simulink library "Flex_Cantilever_Lib"  (R2019b)
settings: Solver=ode45  StartTime=0.0  StopTime=10.0  RelTol=1e-3
undefined symbols (not defined in the file): cantilever_aluminum, fBeamElement, gcbh, mech_rtmsupport, mech_support
libraries: mblibv1 x11, Flex_Cantilever_Element_Lib x9, cstblocks x1, $bdroot x1, SingleDofForceElement x1
Description:
  | Copyright 2009-2017 The MathWorks, Inc. MathWorks, Inc.
settings Model: Creator=smiller  LastModifiedBy=bhisma
settings DataIOCC: LimitDataPoints=on  SaveFormat=Array  SignalLoggingSaveFormat=ModelDataLogs  ReturnWorkspaceOutputs=off
settings OptimizationCC: BlockReduction=off  BooleanDataType=off  ExpressionDepthLimit=2147483647  LifeSpan=inf
settings DebuggingCC: SaveWithParameterizedLinksMsg=none  UnderspecifiedInitializationDetection=Classic  MergeDetectMultiDrivingBlocksExec=none  SignalResolutionControl=TryResolveAllWithWarning  FcnCallInpInsideContextMsg=warning  AllowSymbolicDim=off  StateNameClashWarn=warning  SFUnexpectedBacktrackingDiag=warning  SFNoUnconditionalDefaultTransitionDiag=warning  SFExecutionAtInitializationDiag=none  ArithmeticOperatorsInVariantConditions=warning
settings HardwareCC: ProdBitPerPointer=32  ProdBitPerSizeT=32  ProdBitPerPtrDiffT=32  ProdLargestAtomicFloat=None  ProdIntDivRoundTo=Undefined  ProdEndianess=Unspecified  ProdWordSize=32  ProdHWDeviceType=32-bit Generic  TargetUnknown=on
settings ModelReferenceCC: PropagateSignalLabelsOutOfModel=off
settings SFSimCC: SimUseLocalCustomCode=off  CustomCodeUndefinedFunction=UseInterfaceOnly
settings RTWCC: RTWUseLocalCustomCode=off
settings CodeAppCC: StateflowObjectComments=on
settings GRTTargetCC: TargetLangStandard=C89/C90 (ANSI)  GeneratePreprocessorConditionals=Disable all  CombineOutputUpdateFcns=off  GRTInterface=on
settings ConfigComp: CovMetricSettings=dw  CovHtmlReporting=on  CovSaveCumulativeToWorkspaceVar=on  CovSaveSingleToWorkspaceVar=on  CovExternalEMLEnable=off  CovSFcnEnable=off

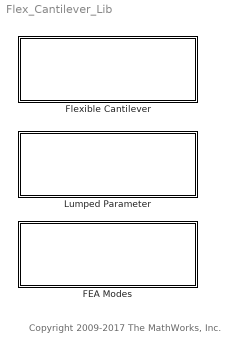
== system Flex_Cantilever_Lib ==
  note: Copyright 2009-2017 The MathWorks, Inc.
  FEA Modes : Subsystem  mask(Cantilever){cantileverData=cantilever_aluminum}
      mask prompts: cantileverData "Cantilever specification"
      mask help:
      | Models a rectangular cross-section cantilever.
      |
      | Specify the name of a cantilever data structure that has the following fields:
      | 	length
      | 	height
      | 	width
      | 	material.density
      | 	material.youngsModulus
      mask init:
      | derivedData = ...
      |     derive_cantilever_properties( cantileverData );
      | L        = derivedData.L;
      | a        = derivedData.a;
      | b        = derivedData.b;
      | volume   = derivedData.volume;
      | mass     = derivedData.mass;
      | inertia  = derivedData.inertia;
      mask Display: image(imread('Flexible_Cantilever_FEA_Beam_IMAGE.jpg'));
  Flexible Cantilever : Subsystem  BlockChoice=FEA Modes
      settings: TemplateBlock=self  MemberBlocks=FEA Modes,Lumped Parameter
  Lumped Parameter : Subsystem
      mask Display: image(imread('Flexible_Cantilever_Lumped_Parameter_IMAGE.jpg'));

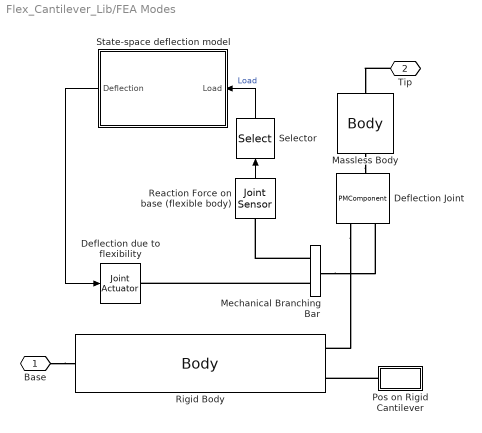
== system Flex_Cantilever_Lib/FEA Modes ==
  Deflection Joint : PMComponent  DialogController=MECH.DynMechDlgSource  LoadFcn=mech_rtmsupport('LoadFcn',gcbh);mech_support('LoadFcn',gcbh);  InitFcn=mech_support('InitFcn');  StartFcn=mech_support('StartFcn',gcbh);  StopFcn=mech_support('StopFcn',gcbh);  PhysicalDomain=mechanical  SubClassName=Unknown  LConnTagsString=__newl0|SA1  RConnTagsString=__newr0  mask(Prismatic){PMImportedID=, NumSAPorts=1, CutJoint=off, MarkAsCut=off, Primitives=prismatic, PrimitiveProps=P1$Base$[0 1 0]$prismatic, ClassName=Joint, DialogClass=JointBlock, P1Axis=[0 1 0]}
      mask prompts: PMImportedID "PMIMPORTED_ID"
      mask help: Represents one translational degree of freedom. The follower (F) body translates relative to the base (B) Body along single translational axis connecting Body coordinate origins. Sensor and actuator ports can be added. Base-follower sequence and axis direction determine sign of forward motion.
      mask init:
      | mech_preinitmask ();
      settings: CopyFcn=mech_rtmsupport('CopyFcn',gcbh);mech_support('CopyFcn',gcbh);  DeleteFcn=mech_rtmsupport('DeleteFcn',gcbh);mech_support('DeleteFcn',gcbh);  UndoDeleteFcn=mech_support('UndoDeleteFcn',gcbh);  ModelCloseFcn=mech_support('ModelCloseFcn',gcbh);  PreSaveFcn=mech_rtmsupport('PreSaveFcn',gcbh);mech_support('PreSaveFcn');  PostSaveFcn=mech_rtmsupport('PostSaveFcn',gcbh);mech_support('PostSaveFcn');  NameChangeFcn=mech_support('NameChangeFcn',gcbh);  PreCopyFcn=mech_rtmsupport('PreCopyFcn',gcbh);  CloseFcn=mech_support('CloseFcn',gcbh);  PreDeleteFcn=mech_rtmsupport('PreDeleteFcn',gcbh);
      mask Help: web(mech_help('prismatic'))
      mask Display: image(mech_getIcon('prismatic.bmp', 'Mechanical'),'center');color('red');text(mech_cutAffordance('offset', gcbh) - 2, 0, mech_cutAffordance('text', gcbh),'HorizontalAlignment', 'right','VerticalAlignment', 'bottom');color('magenta');port_label('LConn', 1, 'B');port_label('RConn', 1, 'F');
  Deflection due to flexibility : mblibv1/Sensors &  Actuators/Joint Actuator  UpdateFromCAD=off  PhysicalDomain=Mechanical  PortType=blob  ActuationStyle=Motion  AngleUnits=deg  ArcVelocityUnits=deg/s  ArcAccelerationUnits=deg/s^2  CoordPositionUnits=m  VelocityUnits=m/s  AccelerationUnits=m/s^2  ForceUnits=N  TorqueUnits=N*m  ActiveIO=off  Width=1  DialogClass=MechanicalActuatorBlock  Primitive=P1  ReferenceFrame=Absolute (World)
      settings: SourceProductName=Simscape Multibody  SourceProductBaseCode=MS
  Massless Body : mblibv1/Bodies/Body  LConnTagsString=CS1  RConnTagsString=CS2  UpdateFromCAD=off  DialogClass=MechanicalBodyBlock  Mass=0  MassUnits=kg  InertiaUnits=kg*m^2  Inertia=eye(3)  Shape=Cylinder  ShapeDims=[1 1]  ShapeUnits=m  ShapeUse=false  Density=1  DensityUnits=kg/m^3  DensityUse=false  GraphicsMode=MACHINE_DEFAULT  BodyColorSelMode=MACHINE_DEFAULT  BodyColor=[1 0 0]  AttachedToCS=CG  CG=Left$CG$[0 0 0]$CS1$CS1$m$[0 0 0]$Euler X-Y-Z$deg$WORLD$false$none  WorkingFrames=Left$CS1$[0 0 0]$Adjoining$Adjoining$m$[0 0 0]$Euler X-Y-Z$deg$WORLD$true$none#Right$CS2$[0 0 0]$CG$CG$m$[0 0 0]$Euler X-Y-Z$deg$WORLD$true$none  CGPos=[0 0 0]  CGRot=[0 0 0]  CS0Pos=[]  CS0Rot=[]  CS1Pos=[0 0 0]  CS1Rot=[0 0 0]  CS2Pos=[0 0 0]  CS2Rot=[0 0 0]  CS3Pos=[]  CS3Rot=[]  CS4Pos=[]  CS4Rot=[]  CS5Pos=[]  CS5Rot=[]  CS6Pos=[]  CS6Rot=[]  CS7Pos=[]  CS7Rot=[]  CS8Pos=[]  CS8Rot=[]  CS9Pos=[]  CS9Rot=[]  CS10Pos=[]  CS10Rot=[]  CS11Pos=[]  CS11Rot=[]  CS12Pos=[]  CS12Rot=[]  CS13Pos=[]  CS13Rot=[]  CS14Pos=[]  CS14Rot=[]  CS15Pos=[]  CS15Rot=[]  CS16Pos=[]  CS16Rot=[]  CS17Pos=[]  CS17Rot=[]  CS18Pos=[]  CS18Rot=[]  CS19Pos=[]  CS19Rot=[]  CS20Pos=[]  CS20Rot=[]
      settings: SourceProductName=Simscape Multibody  SourceProductBaseCode=MS
  Mechanical Branching Bar : mblibv1/Utilities/Mechanical Branching Bar  LConnTagsString=_newl0  RConnTagsString=SA0|SA1  UpdateFromCAD=off  DialogClass=MechanicalBranchingBarBlock  NumSAPorts=2
      settings: SourceProductName=Simscape Multibody  SourceProductBaseCode=MS
  Pos on Rigid Cantilever : Subsystem
  Reaction Force on base (flexible body) : mblibv1/Sensors &  Actuators/Joint Sensor  UpdateFromCAD=off  PhysicalDomain=Mechanical  PortType=blob  Muxed=on  Pose=off  Angle=on  AngleUnits=deg  ArcVelocity=off  ArcVelocityUnits=deg/s  ArcAcceleration=off  ArcAccelerationUnits=deg/s^2  CoordPosition=off  CoordPositionUnits=m  Velocity=off  VelocityUnits=m/s  Acceleration=off  AccelerationUnits=m/s^2  Quaternion=on  QuaternionDT=off  QuaternionDDT=off  QuaternionUnits=off  OutputVector=[1]  ActiveIO=off  Width=1  DialogClass=MechanicalSensorBlock  Primitive=P1  Force=off  ForceUnits=N  Torque=off  TorqueUnits=N*m  ReferenceFrame=Absolute (World)  ReactionSensedSide=Base  ReactionReferenceFrame=Local (Body CS)  ReactionForce=on  ReactionForceUnits=N  ReactionMoment=off  ReactionMomentUnits=N*m
      settings: SourceProductName=Simscape Multibody  SourceProductBaseCode=MS
  Rigid Body : mblibv1/Bodies/Body  LConnTagsString=CS1  RConnTagsString=CS6|CS8  UpdateFromCAD=off  DialogClass=MechanicalBodyBlock  Mass=mass  MassUnits=kg  InertiaUnits=kg*m^2  Inertia=inertia  Shape=Cylinder  ShapeDims=[1 1]  ShapeUnits=m  ShapeUse=false  Density=1  DensityUnits=kg/m^3  DensityUse=false  GraphicsMode=1  BodyColorSelMode=MACHINE_DEFAULT  BodyColor=[0.5 0.5 0.5]  AttachedToCS=1  CG=Left$CG$[L/2 0 0]$CS1$CS1$m$[0 0 0]$Euler X-Y-Z$deg$CS1$false$none  WorkingFrames=Left$CS1$[0 0 0]$Adjoining$Adjoining$m$[0 0 0]$Euler X-Y-Z$deg$Adjoining$true$none#Right$CS2$[0 a b]$CS1$CS1$m$[0 0 0]$Euler X-Y-Z$deg$CS1$false$none#Right$CS3$[0 a -b]$CS1$CS1$m$[0 0 0]$Euler X-Y-Z$deg$CS1$false$none#Right$CS5$[0 -a b]$CS1$CS1$m$[0 0 0]$Euler X-Y-Z$deg$CS1$false$none#Right$CS4$[0 -a -b]$CS1$CS1$m$[0 0 0]$Euler X-Y-Z$deg$CS1$false$none#Right$CS6$[L/2 0 0]$CG$CG$m$[0 0 0]$Euler X-Y-Z$deg$CS1$true$none#Right$CS7$[0 a b]$CS6$CS6$m$[0 0 0]$Euler X-Y-Z$deg$CS1$false$none#Right$CS10$[0 a -b]$CS6$CS6$m$[0 0 0]$Euler X-Y-Z$deg$CS1$false$none#Right$CS9$[0 -a b]$CS6$CS6$m$[0 0 0]$Euler X-Y-Z$deg$CS1$false$none#Right$CS8$[0 -a -b]$CS6$CS6$m$[0 0 0]$Euler X-Y-Z$deg$CS1$true$none  CGPos=[L/2 0 0]  CGRot=[0 0 0]  CS0Pos=[]  CS0Rot=[]  CS1Pos=[0 0 0]  CS1Rot=[0 0 0]  CS2Pos=[0 a b]  CS2Rot=[0 0 0]  CS3Pos=[0 a -b]  CS3Rot=[0 0 0]  CS4Pos=[0 -a -b]  CS4Rot=[0 0 0]  CS5Pos=[0 -a b]  CS5Rot=[0 0 0]  CS6Pos=[L/2 0 0]  CS6Rot=[0 0 0]  CS7Pos=[0 a b]  CS7Rot=[0 0 0]  CS8Pos=[0 -a -b]  CS8Rot=[0 0 0]  CS9Pos=[0 -a b]  CS9Rot=[0 0 0]  CS10Pos=[0 a -b]  CS10Rot=[0 0 0]  CS11Pos=[]  CS11Rot=[]  CS12Pos=[]  CS12Rot=[]  CS13Pos=[]  CS13Rot=[]  CS14Pos=[]  CS14Rot=[]  CS15Pos=[]  CS15Rot=[]  CS16Pos=[]  CS16Rot=[]  CS17Pos=[]  CS17Rot=[]  CS18Pos=[]  CS18Rot=[]  CS19Pos=[]  CS19Rot=[]  CS20Pos=[]  CS20Rot=[]
      settings: SourceProductName=Simscape Multibody  SourceProductBaseCode=MS
  Selector : Selector  InputPortWidth=3  IndexOptions=Index vector (dialog)  Indices=[2]  OutputSizes=1
  State-space deflection model : Subsystem
  Base : PMIOPort  Side=Left
  Tip : PMIOPort  Port=2  Side=Right
  wires:
  Selector/1 -> State-space deflection model/1(Load)  "Load"
  Reaction Force on base (flexible body)/1 -> Selector/1
  State-space deflection model/1(Deflection) -> Deflection due to flexibility/1
  connections:
  Tip/RConn1 -- Massless Body/RConn1
  Deflection Joint/LConn1 -- Rigid Body/RConn1
  Base/RConn1 -- Rigid Body/LConn1
  Pos on Rigid Cantilever/LConn1 -- Rigid Body/RConn2
  Massless Body/LConn1 -- Deflection Joint/RConn1
  Mechanical Branching Bar/RConn1 -- Reaction Force on base (flexible body)/LConn1
  Mechanical Branching Bar/LConn1 -- Deflection Joint/LConn2
  Mechanical Branching Bar/RConn2 -- Deflection due to flexibility/RConn1

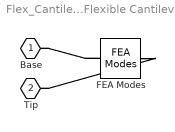
== system Flex_Cantilever_Lib/Flexible Cantilever ==
  FEA Modes : $bdroot/FEA Modes  cantileverData=cantilever_aluminum
  Base : PMIOPort  Side=Left
  Tip : PMIOPort  Port=2  Side=Right
  connections:
  FEA Modes/LConn1 -- Base/RConn1
  FEA Modes/RConn1 -- Tip/RConn1

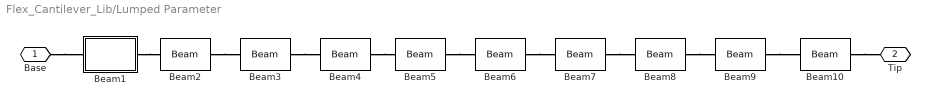
== system Flex_Cantilever_Lib/Lumped Parameter ==
  Beam1 : Subsystem
  Beam{2..10} (9 alike) : Flex_Cantilever_Element_Lib/Beam
  Base : PMIOPort  Side=Left
  Tip : PMIOPort  Port=2  Side=Right
  connections:
  Beam10/RConn1 -- Tip/RConn1
  Base/RConn1 -- Beam1/LConn1
  Beam5/RConn1 -- Beam6/LConn1
  Beam3/RConn1 -- Beam4/LConn1
  Beam2/RConn1 -- Beam3/LConn1
  Beam7/RConn1 -- Beam8/LConn1
  Beam1/RConn1 -- Beam2/LConn1
  Beam9/RConn1 -- Beam10/LConn1
  Beam8/RConn1 -- Beam9/LConn1
  Beam4/RConn1 -- Beam5/LConn1
  Beam6/RConn1 -- Beam7/LConn1

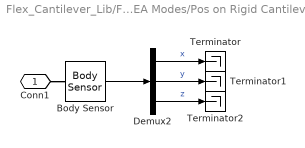
== system Flex_Cantilever_Lib/FEA Modes/Pos on Rigid Cantilever ==
  Body Sensor : mblibv1/Sensors &  Actuators/Body Sensor  UpdateFromCAD=off  PhysicalDomain=Mechanical  PortType=blob  Muxed=on  Pose=off  Angle=on  AngleUnits=deg  ArcVelocity=off  ArcVelocityUnits=deg/s  ArcAcceleration=off  ArcAccelerationUnits=deg/s^2  CoordPosition=on  CoordPositionUnits=m  Velocity=off  VelocityUnits=m/s  Acceleration=off  AccelerationUnits=m/s^2  Quaternion=on  QuaternionDT=off  QuaternionDDT=off  QuaternionUnits=off  OutputVector=[1]  ActiveIO=off  Width=3  DialogClass=MechanicalSensorBlock  ReferenceFrame=Absolute (World)
      settings: SourceProductName=Simscape Multibody  SourceProductBaseCode=MS
  Demux2 : Demux  Outputs=3
  Terminator : Terminator
  Terminator1 : Terminator
  Terminator2 : Terminator
  Conn1 : PMIOPort  Side=Left
  wires:
  Body Sensor/1 -> Demux2/1
  Demux2/1 -> Terminator/1  "x"
  Demux2/2 -> Terminator1/1  "y"
  Demux2/3 -> Terminator2/1  "z"
  connections:
  Conn1/RConn1 -- Body Sensor/LConn1

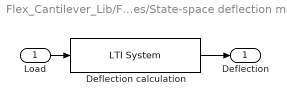
== system Flex_Cantilever_Lib/FEA Modes/State-space deflection model ==
  Load : Inport
  Deflection calculation : cstblocks/LTI System  sys=ss_cantilever_pva  IC=[]
  Deflection : Outport
  wires:
  Load/1 -> Deflection calculation/1
  Deflection calculation/1 -> Deflection/1

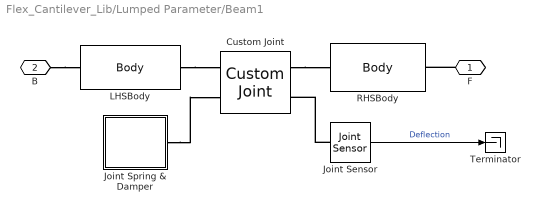
== system Flex_Cantilever_Lib/Lumped Parameter/Beam1 ==
  Custom Joint : mblibv1/Joints/Custom Joint  LConnTagsString=__newl0|SA1  RConnTagsString=__newr0|SA1  UpdateFromCAD=off  NumSAPorts=2  CutJoint=off  MarkAsCut=off  Primitives=revolute  PrimitiveProps=R1$Base$[0 0 1]$Revolute  DialogClass=JointBlock  R1Axis=[0 0 1]  R2Axis=[]  R3Axis=[]  P1Axis=[]  P2Axis=[]  P3Axis=[]  SAxis=[]
      settings: SourceProductName=Simscape Multibody  SourceProductBaseCode=MS
  Joint Sensor : mblibv1/Sensors &  Actuators/Joint Sensor  UpdateFromCAD=off  PhysicalDomain=Mechanical  PortType=blob  Muxed=off  Pose=off  Angle=on  AngleUnits=rad  ArcVelocity=off  ArcVelocityUnits=rad/s  ArcAcceleration=off  ArcAccelerationUnits=deg/s^2  CoordPosition=on  CoordPositionUnits=m  Velocity=off  VelocityUnits=m/s  Acceleration=off  AccelerationUnits=m/s^2  Quaternion=on  QuaternionDT=off  QuaternionDDT=off  QuaternionUnits=off  OutputVector=[1]  ActiveIO=off  Width=1  DialogClass=MechanicalSensorBlock  Primitive=R1  Force=off  ForceUnits=N  Torque=off  TorqueUnits=N*m  ReferenceFrame=Absolute (World)  ReactionSensedSide=Base  ReactionReferenceFrame=Absolute (World)  ReactionForce=off  ReactionForceUnits=N  ReactionMoment=off  ReactionMomentUnits=N*m
      settings: SourceProductName=Simscape Multibody  SourceProductBaseCode=MS
  Joint Spring & Damper : Subsystem  DialogController=MECH.DynMechDlgSource  LoadFcn=mech_rtmsupport('LoadFcn',gcbh);mech_support('LoadFcn',gcbh);  StartFcn=mech_support('StartFcn',gcbh);  StopFcn=mech_support('StopFcn',gcbh);  mask(Joint Spring & Damper){PMImportedID=, ClassName=JointSpringDamper, DialogClass=JointSpringDamper, JFEParameters=P1$false$0$0$0$m$m/s$N$deg$deg/s$N*m#P2$false$0$0$0$m$m/s$N$deg$deg/s$N*m#P3$false$0$0$0$m$m/s$N$deg$deg/s$N*m#R1$true$fBeamElement.EI/fBeamElement.length$fBeamElement.matDamping$0$m$m/s$N$rad$rad/s$N*m#R2$false$0$0$0$m$m/s$N$deg$deg/s$N*m#R3$false$0$0$0$m$m/s$N$deg$deg/s$N*m#S$false$0$0$0$m$m/s$N$deg$deg/s$N*m}
      mask prompts: PMImportedID "PMIMPORTED_ID"
      mask help: Models a damped linear oscillator in a Joint connecting two Bodies, equivalent to a translational spring and damper on prismatic primitives and a torsional spring and damper on revolute primitives. The force or torque F between the bodies is a function of the relative linear or angular displacement x and the linear or angular velocity v of the bodies, given by F = -k*(x-x0) - b*v. The parameters x0, k, and b represent the spring offset, spring constant, and damper constant, respectively. Each prismatic and revolute primitive has a separate spring.
      mask init:
      | mech_preinitmask ();
      | mech_support('MaskInit', gcbh);
      settings: CopyFcn=mech_rtmsupport('CopyFcn',gcbh);mech_support('CopyFcn',gcbh);  DeleteFcn=mech_rtmsupport('DeleteFcn',gcbh);mech_support('DeleteFcn',gcbh);  UndoDeleteFcn=mech_support('UndoDeleteFcn',gcbh);  ModelCloseFcn=mech_support('ModelCloseFcn',gcbh);  PreSaveFcn=mech_rtmsupport('PreSaveFcn',gcbh);mech_support('PreSaveFcn');  PostSaveFcn=mech_rtmsupport('PostSaveFcn',gcbh);mech_support('PostSaveFcn');  NameChangeFcn=mech_support('NameChangeFcn',gcbh);  PreCopyFcn=mech_rtmsupport('PreCopyFcn',gcbh);  CloseFcn=mech_support('CloseFcn',gcbh);  PreDeleteFcn=mech_rtmsupport('PreDeleteFcn',gcbh);
      mask Help: web(mech_help('jointspringdamper'))
      mask Display: image(mech_getIcon('joint_springdamper.bmp', 'Mechanical'),'center')
  LHSBody : mblibv1/Bodies/Body  LConnTagsString=CS1  RConnTagsString=CS2  UpdateFromCAD=off  DialogClass=MechanicalBodyBlock  Mass=fBeamElement.mass  MassUnits=kg  InertiaUnits=kg*m^2  Inertia=fBeamElement.inertia  Shape=Cylinder  ShapeDims=[1 1]  ShapeUnits=m  ShapeUse=false  Density=1  DensityUnits=kg/m^3  DensityUse=false  GraphicsMode=1  BodyColorSelMode=MACHINE_DEFAULT  BodyColor=[0.5 0.5 0.5]  AttachedToCS=1  CG="Left$CG$[fBeamElement.length  0 0]/4$CS1$CS1$m$[0 0 0]$Euler X-Y-Z$deg$CS1$false$none"  WorkingFrames="Left$CS1$[0 0 0]$Adjoining$Adjoining$m$[0 0 0]$Euler X-Y-Z$deg$Adjoining$true$none#Right$CS2$[fBeamElement.length  0 0]/2$CS1$CS1$m$[0 0 0]$Euler X-Y-Z$deg$CS1$true$none#Left$CS3$[0 0 0]$CG$CG$m$[0 0 0]$Euler X-Y-Z$deg$CS1$false$none#Right$CS4$[0 0 0]$CG$CG$m$[0 0 0]$Euler X-Y-Z$deg$CS1$false$none"  CGPos="[fBeamElement.length  0 0]/4"  CGRot=[0 0 0]  CS0Pos=[]  CS0Rot=[]  CS1Pos=[0 0 0]  CS1Rot=[0 0 0]  CS2Pos="[fBeamElement.length  0 0]/2"  CS2Rot=[0 0 0]  CS3Pos=[0 0 0]  CS3Rot=[0 0 0]  CS4Pos=[0 0 0]  CS4Rot=[0 0 0]  CS5Pos=[]  CS5Rot=[]  CS6Pos=[]  CS6Rot=[]  CS7Pos=[]  CS7Rot=[]  CS8Pos=[]  CS8Rot=[]  CS9Pos=[]  CS9Rot=[]  CS10Pos=[]  CS10Rot=[]  CS11Pos=[]  CS11Rot=[]  CS12Pos=[]  CS12Rot=[]  CS13Pos=[]  CS13Rot=[]  CS14Pos=[]  CS14Rot=[]  CS15Pos=[]  CS15Rot=[]  CS16Pos=[]  CS16Rot=[]  CS17Pos=[]  CS17Rot=[]  CS18Pos=[]  CS18Rot=[]  CS19Pos=[]  CS19Rot=[]  CS20Pos=[]  CS20Rot=[]
      settings: SourceProductName=Simscape Multibody  SourceProductBaseCode=MS
  RHSBody : mblibv1/Bodies/Body  LConnTagsString=CS1  RConnTagsString=CS2  UpdateFromCAD=off  DialogClass=MechanicalBodyBlock  Mass=fBeamElement.mass  MassUnits=kg  InertiaUnits=kg*m^2  Inertia=fBeamElement.inertia  Shape=Cylinder  ShapeDims=[1 1]  ShapeUnits=m  ShapeUse=false  Density=1  DensityUnits=kg/m^3  DensityUse=false  GraphicsMode=1  BodyColorSelMode=MACHINE_DEFAULT  BodyColor=[0.5 0.5 0.5]  AttachedToCS=1  CG="Left$CG$[fBeamElement.length  0 0]/2$CS1$CS1$m$[0 0 0]$Euler X-Y-Z$deg$CS1$false$none"  WorkingFrames="Left$CS1$[0 0 0]$Adjoining$Adjoining$m$[0 0 0]$Euler X-Y-Z$deg$Adjoining$true$none#Right$CS2$[fBeamElement.length  0 0]/2$CS1$CS1$m$[0 0 0]$Euler X-Y-Z$deg$CS1$true$none#Right$CS3$[0 0 0]$CG$CG$m$[0 0 0]$Euler X-Y-Z$deg$CS1$false$none#Left$CS4$[0 0 0]$CG$CG$m$[0 0 0]$Euler X-Y-Z$deg$CS1$false$none"  CGPos="[fBeamElement.length  0 0]/2"  CGRot=[0 0 0]  CS0Pos=[]  CS0Rot=[]  CS1Pos=[0 0 0]  CS1Rot=[0 0 0]  CS2Pos="[fBeamElement.length  0 0]/2"  CS2Rot=[0 0 0]  CS3Pos=[0 0 0]  CS3Rot=[0 0 0]  CS4Pos=[0 0 0]  CS4Rot=[0 0 0]  CS5Pos=[]  CS5Rot=[]  CS6Pos=[]  CS6Rot=[]  CS7Pos=[]  CS7Rot=[]  CS8Pos=[]  CS8Rot=[]  CS9Pos=[]  CS9Rot=[]  CS10Pos=[]  CS10Rot=[]  CS11Pos=[]  CS11Rot=[]  CS12Pos=[]  CS12Rot=[]  CS13Pos=[]  CS13Rot=[]  CS14Pos=[]  CS14Rot=[]  CS15Pos=[]  CS15Rot=[]  CS16Pos=[]  CS16Rot=[]  CS17Pos=[]  CS17Rot=[]  CS18Pos=[]  CS18Rot=[]  CS19Pos=[]  CS19Rot=[]  CS20Pos=[]  CS20Rot=[]
      settings: SourceProductName=Simscape Multibody  SourceProductBaseCode=MS
  Terminator : Terminator
  F : PMIOPort  Side=Right
  B : PMIOPort  Port=2  Side=Left
  wires:
  Joint Sensor/1 -> Terminator/1  "Deflection"
  connections:
  LHSBody/RConn1 -- Custom Joint/LConn1
  Custom Joint/RConn1 -- RHSBody/LConn1
  F/RConn1 -- RHSBody/RConn1
  B/RConn1 -- LHSBody/LConn1
  Joint Spring & Damper/LConn1 -- Custom Joint/LConn2
  Joint Sensor/LConn1 -- Custom Joint/RConn2

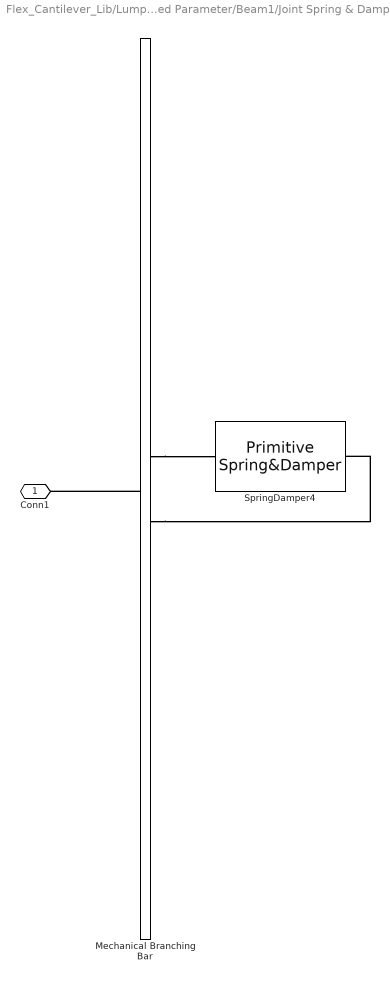
== system Flex_Cantilever_Lib/Lumped Parameter/Beam1/Joint Spring & Damper ==
  Mechanical Branching Bar : mblibv1/Utilities/Mechanical Branching Bar  LConnTagsString=_newl0  RConnTagsString=SA1|SA2|SA3|SA4|SA5|SA6|SA7|SA8|SA9|SA10|SA11|SA12|SA13|SA14  UpdateFromCAD=off  DialogClass=MechanicalBranchingBarBlock  NumSAPorts=14
      settings: SourceProductName=Simscape Multibody  SourceProductBaseCode=MS
  SpringDamper4 : SingleDofForceElement/Primitive Spring&Damper  actuatedPrimitive=R1  springPositionOffset=0  damperVelocityOffset=0  springConstant=fBeamElement.EI/fBeamElement.length  damperConstant=fBeamElement.matDamping  positionUnits=m  angleUnits=rad  velocityUnits=m/s  angleVelocityUnits=rad/s  forceUnits=N  torqueUnits=N*m
      settings: SourceProductName=Simscape Multibody  SourceProductBaseCode=MS
  Conn1 : PMIOPort  Side=Left
  connections:
  Mechanical Branching Bar/LConn1 -- Conn1/RConn1
  Mechanical Branching Bar/RConn7 -- SpringDamper4/LConn1
  Mechanical Branching Bar/RConn8 -- SpringDamper4/RConn1
